simulink model "diskret"  (R2023b)
settings: Solver=VariableStepAuto  StartTime=0.0  StopTime=20  RelTol=1e-3
values from neighbouring files (symbols this model uses):
  Gz_tot = k_r * (Bz / (Az * Cz + Bz * Dz))    [script1.m]
settings Model: Creator=jonatan  LastModifiedBy=jonatan

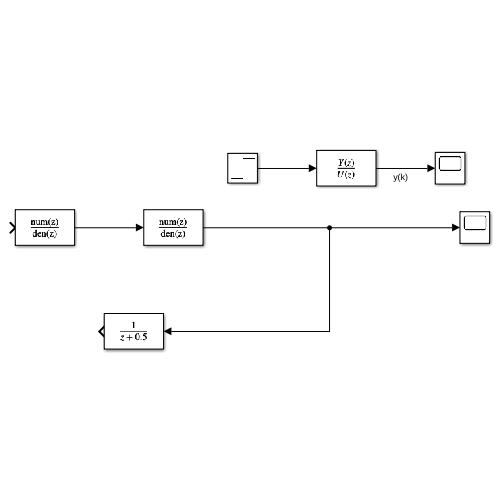
[thumbnail: Simulink's stored preview of the top-level diagram]
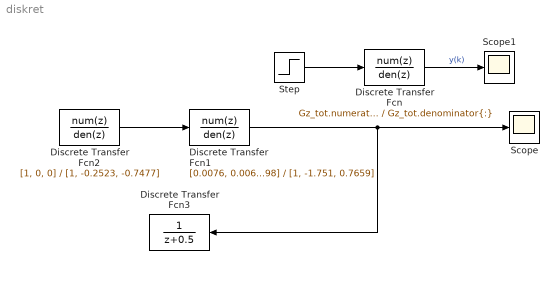
== system diskret ==
  Discrete Transfer Fcn : DiscreteTransferFcn  Numerator=Gz_tot.numerator{:}  Denominator=Gz_tot.denominator{:}
  Discrete Transfer Fcn1 : DiscreteTransferFcn  Numerator=[0.0076, 0.00698]  Denominator=[1, -1.751, 0.7659]
  Discrete Transfer Fcn2 : DiscreteTransferFcn  Numerator=[1, 0, 0]  Denominator=[1, -0.2523, -0.7477]
  Discrete Transfer Fcn3 : DiscreteTransferFcn
  Scope : Scope
  Scope1 : Scope
  Step : Step  SampleTime=1
  wires:
  Discrete Transfer Fcn1/1 -> Discrete Transfer Fcn3/1, Scope/1
  Discrete Transfer Fcn2/1 -> Discrete Transfer Fcn1/1
  Discrete Transfer Fcn/1 -> Scope1/1  "y(k)"
  Step/1 -> Discrete Transfer Fcn/1
